simulink model "c_syntax"  (Simulink 7.6)
settings: Solver=FixedStepDiscrete  StartTime=0.0  StopTime=10.0  FixedStep=1  RelTol=1e-3
PreLoadFcn:
  | busobjectspec
settings Model: Creator=hnine  LastModifiedBy=c2wt
settings DataIOCC: SaveFormat=Structure
settings OptimizationCC: InitFltsAndDblsToZero=on
settings DebuggingCC: SaveWithParameterizedLinksMsg=none  StrictBusMsg=Warning
settings SFSimCC: SimParseCustomCode=off
settings GRTTargetCC: TargetFcnLib=ansi_tfl_tmw.mat

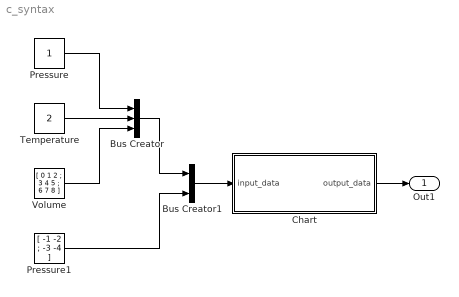
== system c_syntax ==
  Bus Creator : BusCreator  Inputs=3  OutDataTypeStr=Bus: bosecondary  NonVirtualBus=on
  Bus Creator1 : BusCreator  Inputs=2  OutDataTypeStr=Bus: boprimary  NonVirtualBus=on
  Chart : Stateflow chart  TreatAsAtomicUnit=on
  Pressure : Constant  OutDataTypeStr=double
  Pressure1 : Constant  Value=[ -1 -2 ; -3 -4 ]  OutDataTypeStr=double
  Temperature : Constant  Value=2  OutDataTypeStr=single
  Volume : Constant  Value=[ 0 1 2 ; 3 4 5 ; 6 7 8 ]  OutDataTypeStr=uint32
  Out1 : Outport
  wires:
  Pressure/1 -> Bus Creator/1
  Temperature/1 -> Bus Creator/2
  Volume/1 -> Bus Creator/3
  Bus Creator/1 -> Bus Creator1/1
  Pressure1/1 -> Bus Creator1/2
  Bus Creator1/1 -> Chart/1(input_data)
  Chart/1(output_data) -> Out1/1

== stateflow chart Chart ==
  (default) -> (junction 3)
  (junction 3) -> (junction 4) : { output_data = input_data.amatrix[ input_data.environment.Volume[0][1] ][ input_data.environment.Pressure ]; }
  data: input_data input double; output_data output double
